simulink model "new_example1"  (R2016a)
settings: Solver=ode3  StartTime=0.0  StopTime=20  FixedStep=0.001  RelTol=1e-3
settings Model: Creator=user  LastModifiedBy=TOSHIBA
settings DataIOCC: LimitDataPoints=on  SaveFormat=Array  SignalLoggingSaveFormat=ModelDataLogs
settings OptimizationCC: ExpressionDepthLimit=2147483647  InitFltsAndDblsToZero=on
settings DebuggingCC: UnderspecifiedInitializationDetection=Classic  MergeDetectMultiDrivingBlocksExec=none  SolverPrmCheckMsg=warning  FcnCallInpInsideContextMsg=UseLocalSettings  StateNameClashWarn=warning
settings HardwareCC: ProdBitPerPointer=32  ProdLargestAtomicFloat=None  ProdIntDivRoundTo=Undefined  ProdEndianess=Unspecified  ProdWordSize=32  ProdHWDeviceType=32-bit Generic
settings ModelReferenceCC: PropagateSignalLabelsOutOfModel=off
settings GRTTargetCC: GeneratePreprocessorConditionals=Use local settings  CombineOutputUpdateFcns=off  GRTInterface=on
settings ConfigComp: CovModelRefEnable=Off

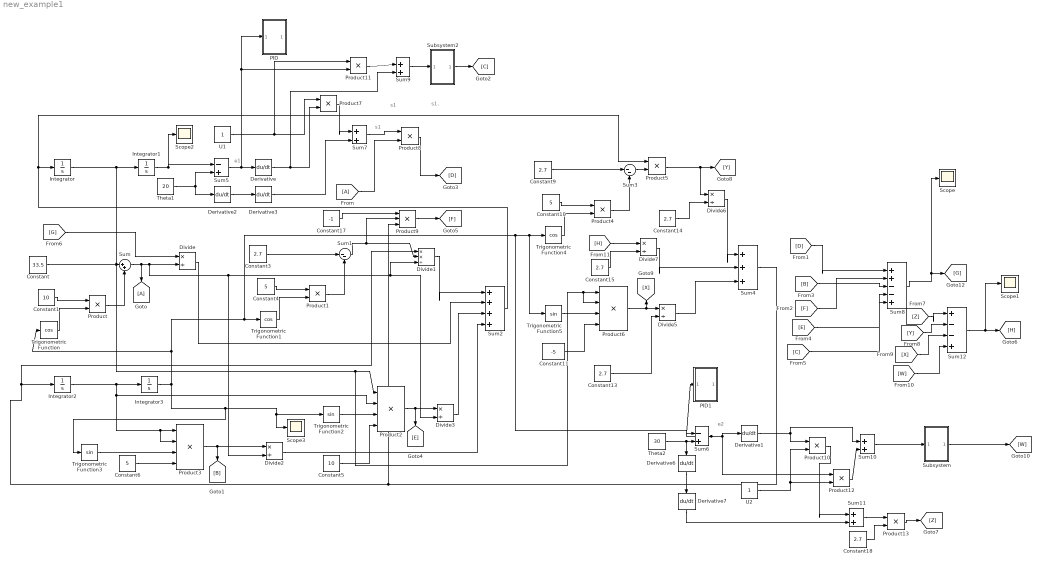
== system new_example1 ==
  note: e1
  note: e2
  note: s1.
  note: s1
  note: s1
  Constant : Constant  Value=33.5
  Constant1 : Constant  Value=10
  Constant10 : Constant  Value=5
  Constant11 : Constant  Value=-5
  Constant{3,9,13..15,18} (6 alike) : Constant  Value=2.7
  Constant17 : Constant  Value=-1
  Constant4 : Constant  Value=5
  Constant5 : Constant  Value=10
  Constant6 : Constant  Value=5
  Derivative{,1..3,6..7} (6 alike) : Derivative
  Divide{,2..3,5..7} (6 alike) : Product  Inputs=*/
  Divide1 : Product  Inputs=**/
  Integrator : Integrator
  Integrator1 : Integrator  InitialCondition=5
  Integrator2 : Integrator
  Integrator3 : Integrator  InitialCondition=-5
  PID : Subsystem
  PID1 : Subsystem
  Product{,1,4..5,7..8,10..13} (10 alike) : Product  RndMeth=Zero
  Product2 : Product  Inputs=4  RndMeth=Zero
  Product3 : Product  Inputs=4  RndMeth=Zero
  Product6 : Product  Inputs=4  RndMeth=Zero
  Product9 : Product  Inputs=3  RndMeth=Zero
  Scope{,1..3} (4 alike) : Scope
  Subsystem : Subsystem
  Subsystem2 : Subsystem
  Sum{,7,9..11} (5 alike) : Sum  Inputs=|++
  Sum1 : Sum  Inputs=|--
  Sum12 : Sum  Inputs=|+--+
  Sum2 : Sum  Inputs=|++++
  Sum3 : Sum  Inputs=|--
  Sum4 : Sum  Inputs=|+++
  Sum5 : Sum  Inputs=|-+
  Sum6 : Sum  Inputs=|-+
  Sum8 : Sum  Inputs=|++--+
  Theta1 : Constant  Value=20
  Theta2 : Constant  Value=30
  Trigonometric Function : Trigonometry  Operator=cos
  Trigonometric Function1 : Trigonometry  Operator=cos
  Trigonometric Function2 : Trigonometry
  Trigonometric Function3 : Trigonometry
  Trigonometric Function4 : Trigonometry  Operator=cos
  Trigonometric Function5 : Trigonometry
  U1 : Constant
  U2 : Constant
  wires:
  Constant1/1 -> Product/1
  Trigonometric Function/1 -> Product/2
  Constant/1 -> Sum/1
  Product/1 -> Sum/2
  Integrator/1 -> Integrator1/1, Product6/2, Product6/1, Product2/1
  Integrator1/1 -> Sum5/1, Scope2/1
  Integrator2/1 -> Product3/1, Product3/2, Product2/2, Integrator3/1
  Integrator3/1 -> Trigonometric Function3/1, Trigonometric Function2/1, Scope3/1, Trigonometric Function/1, Trigonometric Function1/1, Trigonometric Function4/1, Trigonometric Function5/1, Sum6/1
  Sum/1 -> Divide/2, Divide2/2, Divide1/3, Divide3/2, [A]
  [G] -> Divide/1
  Constant4/1 -> Product1/1
  Trigonometric Function1/1 -> Product1/2
  Constant3/1 -> Sum1/1
  Product1/1 -> Sum1/2
  Sum1/1 -> Product9/2, Divide1/2
  Constant5/1 -> Product2/4
  Trigonometric Function2/1 -> Product2/3
  Constant6/1 -> Product3/4
  Trigonometric Function3/1 -> Product3/3
  Product3/1 -> Divide2/1, [B]
  Product2/1 -> Divide3/1, [E]
  Divide1/1 -> Sum2/1
  Divide3/1 -> Sum2/3
  Divide2/1 -> Sum2/4
  Divide/1 -> Sum2/2
  Constant10/1 -> Product4/1
  Trigonometric Function4/1 -> Product4/2
  Constant9/1 -> Sum3/1
  Product4/1 -> Sum3/2
  Sum3/1 -> Product5/2
  Sum2/1 -> Integrator/1, Product5/1
  Constant11/1 -> Product6/4
  Trigonometric Function5/1 -> Product6/3
  Product6/1 -> Divide5/1, [X]
  Constant13/1 -> Divide5/2
  Product5/1 -> Divide6/1, [Y]
  Constant14/1 -> Divide6/2
  [H] -> Divide7/1
  Constant15/1 -> Divide7/2
  Divide7/1 -> Sum4/2
  Divide5/1 -> Sum4/3
  Divide6/1 -> Sum4/1
  Sum4/1 -> Integrator2/1, Divide1/1, Product9/3
  Theta1/1 -> Derivative2/1, Sum5/2
  Sum5/1 -> Derivative/1, Product11/2, PID/1(In1)
  Theta2/1 -> Sum6/2, Derivative6/1
  Sum6/1 -> Derivative1/1, Product12/1, PID1/1(In1)
  Derivative2/1 -> Derivative3/1
  Derivative3/1 -> Sum7/2
  U1/1 -> Product11/1, Product7/1
  Derivative/1 -> Sum9/2, Product7/2
  Product7/1 -> Sum7/1
  [A] -> Product8/2
  Constant17/1 -> Product9/1
  Subsystem2/1(Out1) -> [C]
  Product8/1 -> [D]
  Product9/1 -> [F]
  [D] -> Sum8/1
  [F] -> Sum8/2
  [B] -> Sum8/3
  [E] -> Sum8/4
  [C] -> Sum8/5
  Sum8/1 -> Scope/1, [G]
  U2/1 -> Product10/2, Product12/2
  Product11/1 -> Sum9/1
  Sum9/1 -> Subsystem2/1(In1)
  Sum7/1 -> Product8/1
  Derivative1/1 -> Product10/1, Sum10/1
  Product12/1 -> Sum10/2
  Derivative6/1 -> Derivative7/1
  Derivative7/1 -> Sum11/2
  Product10/1 -> Sum11/1
  Sum11/1 -> Product13/1
  Constant18/1 -> Product13/2
  Product13/1 -> [Z]
  [Z] -> Sum12/1
  [Y] -> Sum12/2
  Sum12/1 -> Scope1/1, [H]
  [X] -> Sum12/3
  [W] -> Sum12/4
  Subsystem/1(Out1) -> [W]
  Sum10/1 -> Subsystem/1(In1)

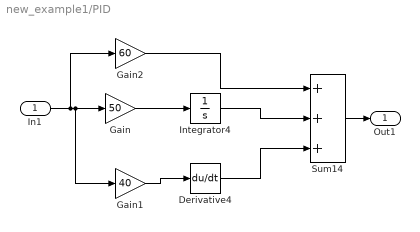
== system new_example1/PID ==
  In1 : Inport
  Derivative4 : Derivative
  Gain : Gain  Gain=50
  Gain1 : Gain  Gain=40
  Gain2 : Gain  Gain=60
  Integrator4 : Integrator
  Sum14 : Sum  Inputs=+++
  Out1 : Outport
  wires:
  Gain/1 -> Integrator4/1
  Gain1/1 -> Derivative4/1
  In1/1 -> Gain1/1, Gain/1, Gain2/1
  Gain2/1 -> Sum14/1
  Integrator4/1 -> Sum14/2
  Derivative4/1 -> Sum14/3
  Sum14/1 -> Out1/1

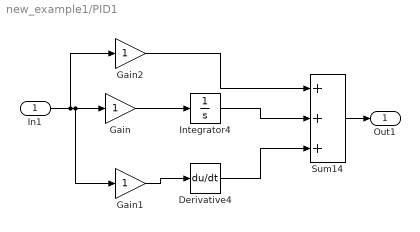
== system new_example1/PID1 ==
  In1 : Inport
  Derivative4 : Derivative
  Gain : Gain
  Gain1 : Gain
  Gain2 : Gain
  Integrator4 : Integrator
  Sum14 : Sum  Inputs=+++
  Out1 : Outport
  wires:
  Sum14/1 -> Out1/1
  Derivative4/1 -> Sum14/3
  Integrator4/1 -> Sum14/2
  Gain2/1 -> Sum14/1
  In1/1 -> Gain2/1, Gain/1, Gain1/1
  Gain1/1 -> Derivative4/1
  Gain/1 -> Integrator4/1

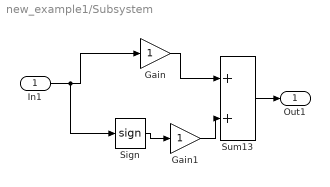
== system new_example1/Subsystem ==
  In1 : Inport
  Gain : Gain
  Gain1 : Gain
  Sign : Signum
  Sum13 : Sum
  Out1 : Outport
  wires:
  Gain/1 -> Sum13/1
  Gain1/1 -> Sum13/2
  Sign/1 -> Gain1/1
  In1/1 -> Sign/1, Gain/1
  Sum13/1 -> Out1/1

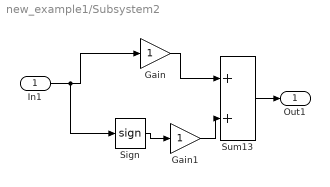
== system new_example1/Subsystem2 ==
  In1 : Inport
  Gain : Gain
  Gain1 : Gain
  Sign : Signum
  Sum13 : Sum
  Out1 : Outport
  wires:
  Gain/1 -> Sum13/1
  Gain1/1 -> Sum13/2
  Sign/1 -> Gain1/1
  In1/1 -> Sign/1, Gain/1
  Sum13/1 -> Out1/1
